simulink model "MPC_backend_matlab"  (R2026a)
settings: Solver=VariableStepAuto
model workspace (MAT data in the model file):
  kappa_ref = 1
  mpc_ref = 1
libraries: mpclib x1
settings Model: Creator=rayyu  LastModifiedBy=rayyu
settings DebuggingCC: UnderSpecifiedDimensionMsg=warning

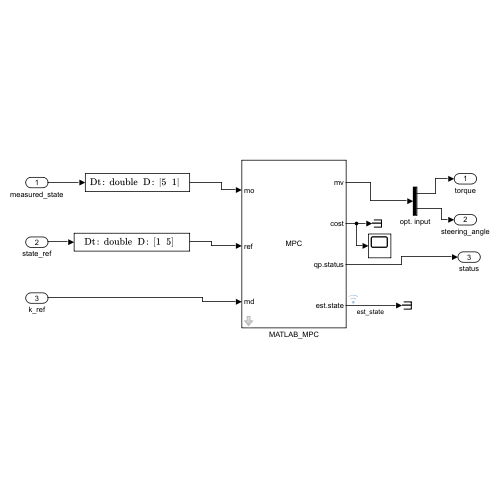
[thumbnail: Simulink's stored preview of the top-level diagram]
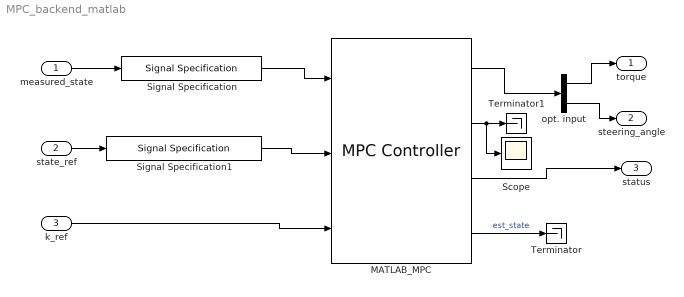
== system MPC_backend_matlab ==
  measured_state : Inport  PortDimensions=5
  state_ref : Inport  Port=2  PortDimensions=[1 5]
  k_ref : Inport  Port=3
  MATLAB_MPC : mpclib/MPC Controller  SCDEnableBlockLinearizationSpecification=on  mpcobj=mpc_baseline  is_multiple=0  enable_value=0  return_u0=off  updateMPCinCallerWorkspace=on  md_inport=on  mv_inport=off  uref_inport=off  return_cost=on  return_mvseq=off  return_qpstatus=on  return_xseq=off  return_state=on  return_ovseq=off  state_inport=off  umin_inport=off  umax_inport=off  ymin_inport=off  ymax_inport=off  cc_inport=off  ywt_inport=off  uwt_inport=off  duwt_inport=off  rhoeps_inport=off  pm_inport=off  MaximumP=10  HorizonChoice=FixedHorizon  n_ts=0.1  n_p=20  n_mv=2  n_md=1  n_ud=0  n_mo=5  n_uo=0  BlockDataType=double  SampleTimeInherited=off  switch_inport=off
  Scope : Scope
      settings: ActiveDisplayYMinimum=-1  ActiveDisplayYMaximum=1
  Signal Specification : SignalSpecification  OutDataTypeStr=double  Dimensions=[5 1]
  Signal Specification1 : SignalSpecification  OutDataTypeStr=double  Dimensions=[1 5]
  Terminator : Terminator
  Terminator1 : Terminator
  opt. input : Demux  Outputs=2
  torque : Outport
  steering_angle : Outport  Port=2
  status : Outport  Port=3
  wires:
  MATLAB_MPC/1 -> opt. input/1
  MATLAB_MPC/3 -> status/1
  measured_state/1 -> Signal Specification/1
  k_ref/1 -> MATLAB_MPC/3
  opt. input/1 -> torque/1
  opt. input/2 -> steering_angle/1
  state_ref/1 -> Signal Specification1/1
  MATLAB_MPC/4 -> Terminator/1  "est_state"
  Signal Specification/1 -> MATLAB_MPC/1
  Signal Specification1/1 -> MATLAB_MPC/2
  MATLAB_MPC/2 -> Scope/1, Terminator1/1
